simulink model "Uby_hinf"  (R2025b)
settings: Solver=VariableStepAuto  StartTime=0.0  StopTime=10.0  RelTol=1e-3
undefined symbols (not defined in the file): A, B_new, C, nu, ny
libraries: cstblocks x2
settings Model: Creator=Miche  LastModifiedBy=Miche

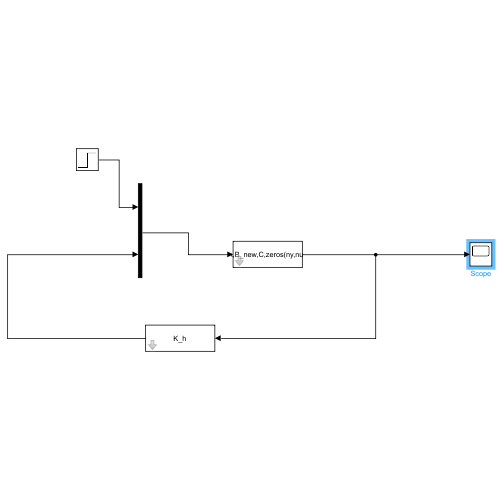
[thumbnail: Simulink's stored preview of the top-level diagram]
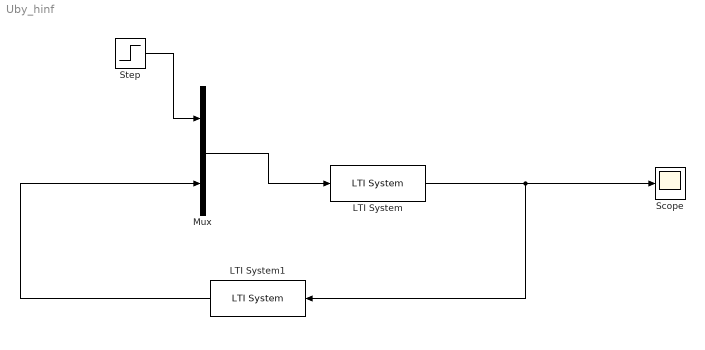
== system Uby_hinf ==
  LTI System : cstblocks/LTI System  sys=ss(A,B_new,C,zeros(ny,nu+1))  IC=h0  PadeOrder=0
  LTI System1 : cstblocks/LTI System  sys=K_h  IC=[]  PadeOrder=0
  Mux : Mux  Inputs=2
  Scope : Scope
      settings: ActiveDisplayYMinimum=-0.24734196560724886  ActiveDisplayYMaximum=0.36081577395636094
  Step : Step  Time=5  After=0.05  SampleTime=0
  wires:
  Mux/1 -> LTI System/1
  LTI System1/1 -> Mux/2
  Step/1 -> Mux/1
  LTI System/1 -> LTI System1/1, Scope/1
